simulink model "Lidar_System_July03"  (Simulink 7.3)
settings: Solver=FixedStepDiscrete  StartTime=0.0  StopTime=inf  FixedStep=0.1  MaxStep=0.2  RelTol=1e-3
undefined symbols (not defined in the file): strel
libraries: dspmtrx3 x88, simulink x65, dspstat3 x37, vipstatistics x15, vipmorphops x15, dspindex x1
(part 2 of 8)

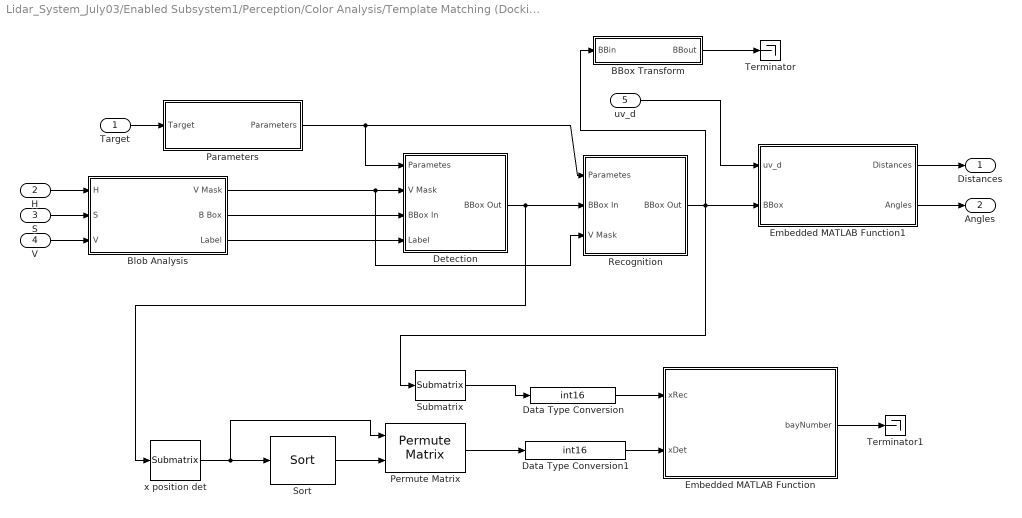
== system Lidar_System_July03/Enabled Subsystem1/Perception/Color Analysis/Template Matching (Docking)/Blue/Circle/Docking1 ==
  Target : Inport
  H : Inport  Port=2
  S : Inport  Port=3
  V : Inport  Port=4
  uv_d : Inport  Port=5
  BBox Transform : Stateflow chart
  Blob Analysis : Subsystem
  Data Type Conversion : DataTypeConversion  OutDataTypeMode=int16  OutDataType=fixdt(1, 16)  OutScaling=2^0  OutDataTypeStr=int16
  Data Type Conversion1 : DataTypeConversion  OutDataTypeMode=int16  OutDataType=fixdt(1, 16)  OutScaling=2^0  OutDataTypeStr=int16
  Detection : Subsystem
  Embedded MATLAB Function : Stateflow chart
  Embedded MATLAB Function1 : Stateflow chart
  Parameters : Subsystem
  Permute Matrix : dspmtrx3/Permute Matrix  mode=Rows  ZeroOneIdxMode=One-based  errmode=Clip index  checkDims=off
  Recognition : Subsystem
  Sort : dspstat3/Sort  DialogController=dspDDGCreate  DialogControllerArgs=DataTag18  otype=Index  dir=Ascending  sortAlg=Quick sort  roundingMode=Floor  overflowMode=off
  Submatrix : dspmtrx3/Submatrix  RowSpan=Range of rows  RowStartMode=First  RowStartIndex=1  RowEndMode=Last  RowEndIndex=1  ColSpan=One column  ColStartMode=First  ColStartIndex=1  ColEndMode=Last  ColEndIndex=1
  Terminator : Terminator
  Terminator1 : Terminator
  x position det : dspmtrx3/Submatrix  RowSpan=Range of rows  RowStartMode=First  RowStartIndex=1  RowEndMode=Last  RowEndIndex=1  ColSpan=One column  ColStartMode=First  ColStartIndex=1  ColEndMode=Last  ColEndIndex=1
  Distances : Outport
  Angles : Outport  Port=2
  wires:
  Embedded MATLAB Function1/2(Angles) -> Angles/1
  BBox Transform/1(BBout) -> Terminator/1
  Target/1 -> Parameters/1(Target)
  V/1 -> Blob Analysis/3(V)
  S/1 -> Blob Analysis/2(S)
  H/1 -> Blob Analysis/1(H)
  Embedded MATLAB Function1/1(Distances) -> Distances/1
  uv_d/1 -> Embedded MATLAB Function1/1(uv_d)
  Embedded MATLAB Function/1(bayNumber) -> Terminator1/1
  Recognition/1(BBox Out) -> BBox Transform/1(BBin), Embedded MATLAB Function1/2(BBox), Submatrix/1
  Data Type Conversion1/1 -> Embedded MATLAB Function/2(xDet)
  Data Type Conversion/1 -> Embedded MATLAB Function/1(xRec)
  Permute Matrix/1 -> Data Type Conversion1/1
  Submatrix/1 -> Data Type Conversion/1
  Sort/1 -> Permute Matrix/2
  x position det/1 -> Permute Matrix/1, Sort/1
  Detection/1(BBox Out) -> x position det/1, Recognition/2(BBox In)
  Blob Analysis/3(Label) -> Detection/4(Label)
  Blob Analysis/2(B Box) -> Detection/3(BBox In)
  Blob Analysis/1(V Mask) -> Recognition/3(V Mask), Detection/2(V Mask)
  Parameters/1(Parameters) -> Recognition/1(Parametes), Detection/1(Parametes)

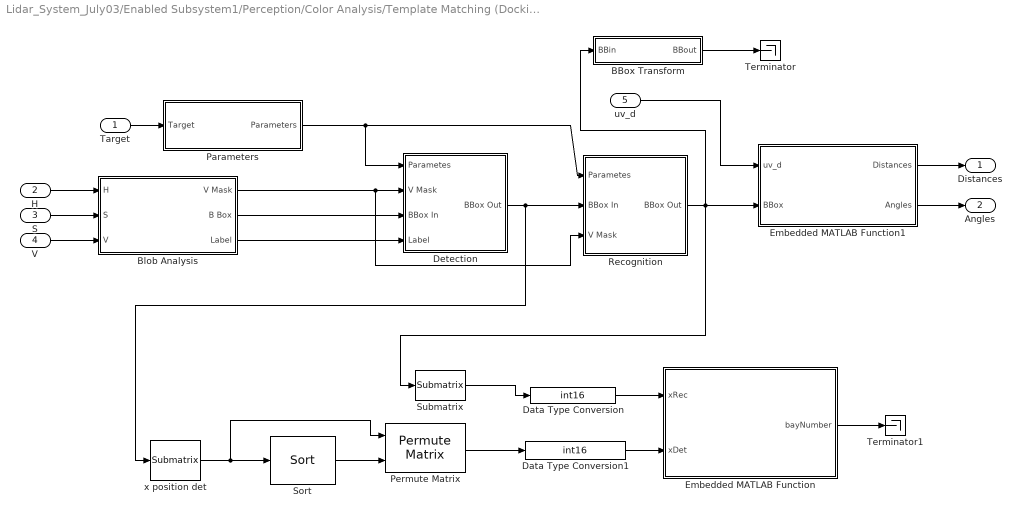
== system Lidar_System_July03/Enabled Subsystem1/Perception/Color Analysis/Template Matching (Docking)/Blue/Cruciform/Docking1 ==
  Target : Inport
  H : Inport  Port=2
  S : Inport  Port=3
  V : Inport  Port=4
  uv_d : Inport  Port=5
  BBox Transform : Stateflow chart
  Blob Analysis : Subsystem
  Data Type Conversion : DataTypeConversion  OutDataTypeMode=int16  OutDataType=fixdt(1, 16)  OutScaling=2^0  OutDataTypeStr=int16
  Data Type Conversion1 : DataTypeConversion  OutDataTypeMode=int16  OutDataType=fixdt(1, 16)  OutScaling=2^0  OutDataTypeStr=int16
  Detection : Subsystem
  Embedded MATLAB Function : Stateflow chart
  Embedded MATLAB Function1 : Stateflow chart
  Parameters : Subsystem
  Permute Matrix : dspmtrx3/Permute Matrix  mode=Rows  ZeroOneIdxMode=One-based  errmode=Clip index  checkDims=off
  Recognition : Subsystem
  Sort : dspstat3/Sort  DialogController=dspDDGCreate  DialogControllerArgs=DataTag22  otype=Index  dir=Ascending  sortAlg=Quick sort  roundingMode=Floor  overflowMode=off
  Submatrix : dspmtrx3/Submatrix  RowSpan=Range of rows  RowStartMode=First  RowStartIndex=1  RowEndMode=Last  RowEndIndex=1  ColSpan=One column  ColStartMode=First  ColStartIndex=1  ColEndMode=Last  ColEndIndex=1
  Terminator : Terminator
  Terminator1 : Terminator
  x position det : dspmtrx3/Submatrix  RowSpan=Range of rows  RowStartMode=First  RowStartIndex=1  RowEndMode=Last  RowEndIndex=1  ColSpan=One column  ColStartMode=First  ColStartIndex=1  ColEndMode=Last  ColEndIndex=1
  Distances : Outport
  Angles : Outport  Port=2
  wires:
  Embedded MATLAB Function1/2(Angles) -> Angles/1
  BBox Transform/1(BBout) -> Terminator/1
  Target/1 -> Parameters/1(Target)
  V/1 -> Blob Analysis/3(V)
  S/1 -> Blob Analysis/2(S)
  H/1 -> Blob Analysis/1(H)
  Embedded MATLAB Function1/1(Distances) -> Distances/1
  uv_d/1 -> Embedded MATLAB Function1/1(uv_d)
  Embedded MATLAB Function/1(bayNumber) -> Terminator1/1
  Recognition/1(BBox Out) -> BBox Transform/1(BBin), Embedded MATLAB Function1/2(BBox), Submatrix/1
  Data Type Conversion1/1 -> Embedded MATLAB Function/2(xDet)
  Data Type Conversion/1 -> Embedded MATLAB Function/1(xRec)
  Permute Matrix/1 -> Data Type Conversion1/1
  Submatrix/1 -> Data Type Conversion/1
  Sort/1 -> Permute Matrix/2
  x position det/1 -> Permute Matrix/1, Sort/1
  Detection/1(BBox Out) -> x position det/1, Recognition/2(BBox In)
  Blob Analysis/3(Label) -> Detection/4(Label)
  Blob Analysis/2(B Box) -> Detection/3(BBox In)
  Blob Analysis/1(V Mask) -> Recognition/3(V Mask), Detection/2(V Mask)
  Parameters/1(Parameters) -> Recognition/1(Parametes), Detection/1(Parametes)

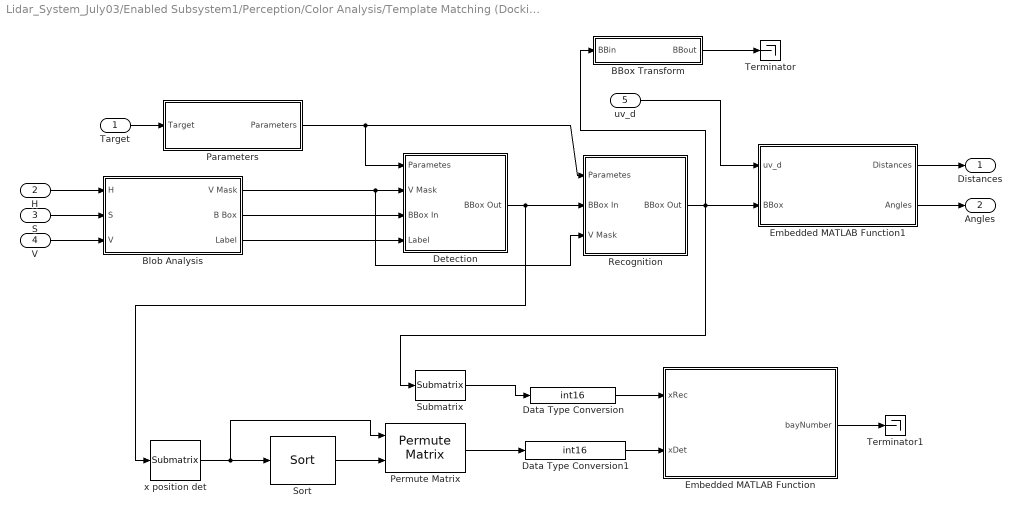
== system Lidar_System_July03/Enabled Subsystem1/Perception/Color Analysis/Template Matching (Docking)/Blue/Triangle/Docking1 ==
  Target : Inport
  H : Inport  Port=2
  S : Inport  Port=3
  V : Inport  Port=4
  uv_d : Inport  Port=5
  BBox Transform : Stateflow chart
  Blob Analysis : Subsystem
  Data Type Conversion : DataTypeConversion  OutDataTypeMode=int16  OutDataType=fixdt(1, 16)  OutScaling=2^0  OutDataTypeStr=int16
  Data Type Conversion1 : DataTypeConversion  OutDataTypeMode=int16  OutDataType=fixdt(1, 16)  OutScaling=2^0  OutDataTypeStr=int16
  Detection : Subsystem
  Embedded MATLAB Function : Stateflow chart
  Embedded MATLAB Function1 : Stateflow chart
  Parameters : Subsystem
  Permute Matrix : dspmtrx3/Permute Matrix  mode=Rows  ZeroOneIdxMode=One-based  errmode=Clip index  checkDims=off
  Recognition : Subsystem
  Sort : dspstat3/Sort  DialogController=dspDDGCreate  DialogControllerArgs=DataTag26  otype=Index  dir=Ascending  sortAlg=Quick sort  roundingMode=Floor  overflowMode=off
  Submatrix : dspmtrx3/Submatrix  RowSpan=Range of rows  RowStartMode=First  RowStartIndex=1  RowEndMode=Last  RowEndIndex=1  ColSpan=One column  ColStartMode=First  ColStartIndex=1  ColEndMode=Last  ColEndIndex=1
  Terminator : Terminator
  Terminator1 : Terminator
  x position det : dspmtrx3/Submatrix  RowSpan=Range of rows  RowStartMode=First  RowStartIndex=1  RowEndMode=Last  RowEndIndex=1  ColSpan=One column  ColStartMode=First  ColStartIndex=1  ColEndMode=Last  ColEndIndex=1
  Distances : Outport
  Angles : Outport  Port=2
  wires:
  Embedded MATLAB Function1/2(Angles) -> Angles/1
  BBox Transform/1(BBout) -> Terminator/1
  Target/1 -> Parameters/1(Target)
  V/1 -> Blob Analysis/3(V)
  S/1 -> Blob Analysis/2(S)
  H/1 -> Blob Analysis/1(H)
  Embedded MATLAB Function1/1(Distances) -> Distances/1
  uv_d/1 -> Embedded MATLAB Function1/1(uv_d)
  Embedded MATLAB Function/1(bayNumber) -> Terminator1/1
  Recognition/1(BBox Out) -> BBox Transform/1(BBin), Embedded MATLAB Function1/2(BBox), Submatrix/1
  Data Type Conversion1/1 -> Embedded MATLAB Function/2(xDet)
  Data Type Conversion/1 -> Embedded MATLAB Function/1(xRec)
  Permute Matrix/1 -> Data Type Conversion1/1
  Submatrix/1 -> Data Type Conversion/1
  Sort/1 -> Permute Matrix/2
  x position det/1 -> Permute Matrix/1, Sort/1
  Detection/1(BBox Out) -> x position det/1, Recognition/2(BBox In)
  Blob Analysis/3(Label) -> Detection/4(Label)
  Blob Analysis/2(B Box) -> Detection/3(BBox In)
  Blob Analysis/1(V Mask) -> Recognition/3(V Mask), Detection/2(V Mask)
  Parameters/1(Parameters) -> Recognition/1(Parametes), Detection/1(Parametes)

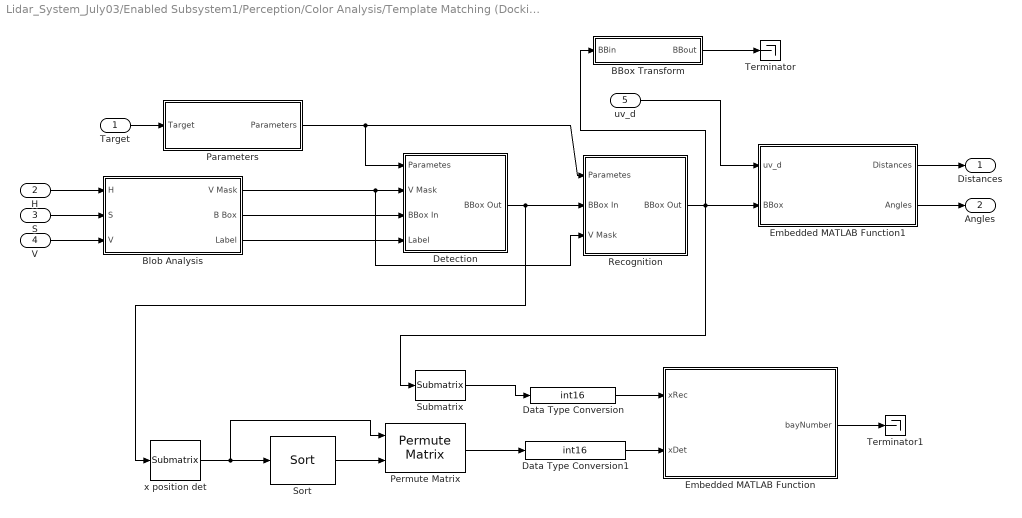
== system Lidar_System_July03/Enabled Subsystem1/Perception/Color Analysis/Template Matching (Docking)/Green/Circle/Docking1 ==
  Target : Inport
  H : Inport  Port=2
  S : Inport  Port=3
  V : Inport  Port=4
  uv_d : Inport  Port=5
  BBox Transform : Stateflow chart
  Blob Analysis : Subsystem
  Data Type Conversion : DataTypeConversion  OutDataTypeMode=int16  OutDataType=fixdt(1, 16)  OutScaling=2^0  OutDataTypeStr=int16
  Data Type Conversion1 : DataTypeConversion  OutDataTypeMode=int16  OutDataType=fixdt(1, 16)  OutScaling=2^0  OutDataTypeStr=int16
  Detection : Subsystem
  Embedded MATLAB Function : Stateflow chart
  Embedded MATLAB Function1 : Stateflow chart
  Parameters : Subsystem
  Permute Matrix : dspmtrx3/Permute Matrix  mode=Rows  ZeroOneIdxMode=One-based  errmode=Clip index  checkDims=off
  Recognition : Subsystem
  Sort : dspstat3/Sort  DialogController=dspDDGCreate  DialogControllerArgs=DataTag30  otype=Index  dir=Ascending  sortAlg=Quick sort  roundingMode=Floor  overflowMode=off
  Submatrix : dspmtrx3/Submatrix  RowSpan=Range of rows  RowStartMode=First  RowStartIndex=1  RowEndMode=Last  RowEndIndex=1  ColSpan=One column  ColStartMode=First  ColStartIndex=1  ColEndMode=Last  ColEndIndex=1
  Terminator : Terminator
  Terminator1 : Terminator
  x position det : dspmtrx3/Submatrix  RowSpan=Range of rows  RowStartMode=First  RowStartIndex=1  RowEndMode=Last  RowEndIndex=1  ColSpan=One column  ColStartMode=First  ColStartIndex=1  ColEndMode=Last  ColEndIndex=1
  Distances : Outport
  Angles : Outport  Port=2
  wires:
  Embedded MATLAB Function1/2(Angles) -> Angles/1
  BBox Transform/1(BBout) -> Terminator/1
  Target/1 -> Parameters/1(Target)
  V/1 -> Blob Analysis/3(V)
  S/1 -> Blob Analysis/2(S)
  H/1 -> Blob Analysis/1(H)
  Embedded MATLAB Function1/1(Distances) -> Distances/1
  uv_d/1 -> Embedded MATLAB Function1/1(uv_d)
  Embedded MATLAB Function/1(bayNumber) -> Terminator1/1
  Recognition/1(BBox Out) -> BBox Transform/1(BBin), Embedded MATLAB Function1/2(BBox), Submatrix/1
  Data Type Conversion1/1 -> Embedded MATLAB Function/2(xDet)
  Data Type Conversion/1 -> Embedded MATLAB Function/1(xRec)
  Permute Matrix/1 -> Data Type Conversion1/1
  Submatrix/1 -> Data Type Conversion/1
  Sort/1 -> Permute Matrix/2
  x position det/1 -> Permute Matrix/1, Sort/1
  Detection/1(BBox Out) -> x position det/1, Recognition/2(BBox In)
  Blob Analysis/3(Label) -> Detection/4(Label)
  Blob Analysis/2(B Box) -> Detection/3(BBox In)
  Blob Analysis/1(V Mask) -> Recognition/3(V Mask), Detection/2(V Mask)
  Parameters/1(Parameters) -> Recognition/1(Parametes), Detection/1(Parametes)

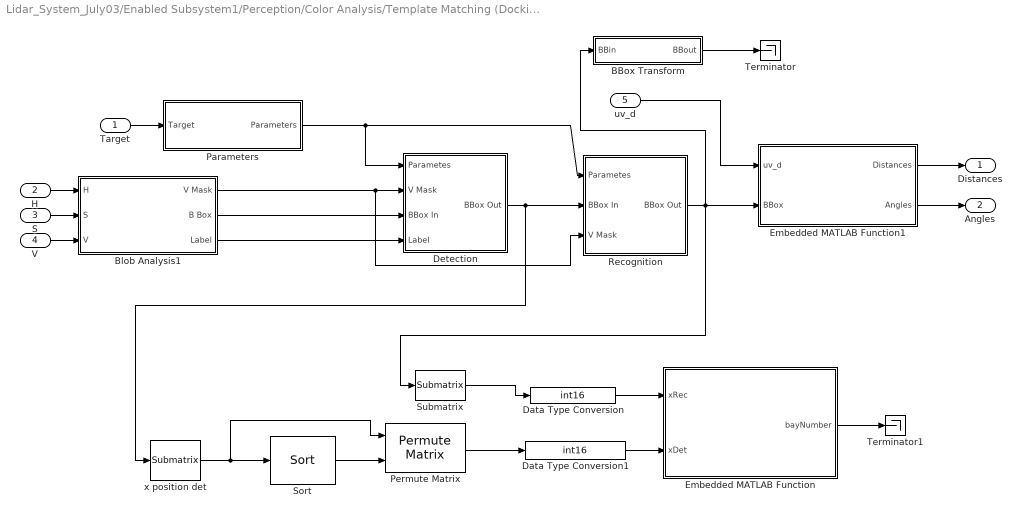
== system Lidar_System_July03/Enabled Subsystem1/Perception/Color Analysis/Template Matching (Docking)/Green/Cruciform/Docking1 ==
  Target : Inport
  H : Inport  Port=2
  S : Inport  Port=3
  V : Inport  Port=4
  uv_d : Inport  Port=5
  BBox Transform : Stateflow chart
  Blob Analysis1 : Subsystem
  Data Type Conversion : DataTypeConversion  OutDataTypeMode=int16  OutDataType=fixdt(1, 16)  OutScaling=2^0  OutDataTypeStr=int16
  Data Type Conversion1 : DataTypeConversion  OutDataTypeMode=int16  OutDataType=fixdt(1, 16)  OutScaling=2^0  OutDataTypeStr=int16
  Detection : Subsystem
  Embedded MATLAB Function : Stateflow chart
  Embedded MATLAB Function1 : Stateflow chart
  Parameters : Subsystem
  Permute Matrix : dspmtrx3/Permute Matrix  mode=Rows  ZeroOneIdxMode=One-based  errmode=Clip index  checkDims=off
  Recognition : Subsystem
  Sort : dspstat3/Sort  DialogController=dspDDGCreate  DialogControllerArgs=DataTag34  otype=Index  dir=Ascending  sortAlg=Quick sort  roundingMode=Floor  overflowMode=off
  Submatrix : dspmtrx3/Submatrix  RowSpan=Range of rows  RowStartMode=First  RowStartIndex=1  RowEndMode=Last  RowEndIndex=1  ColSpan=One column  ColStartMode=First  ColStartIndex=1  ColEndMode=Last  ColEndIndex=1
  Terminator : Terminator
  Terminator1 : Terminator
  x position det : dspmtrx3/Submatrix  RowSpan=Range of rows  RowStartMode=First  RowStartIndex=1  RowEndMode=Last  RowEndIndex=1  ColSpan=One column  ColStartMode=First  ColStartIndex=1  ColEndMode=Last  ColEndIndex=1
  Distances : Outport
  Angles : Outport  Port=2
  wires:
  Embedded MATLAB Function1/2(Angles) -> Angles/1
  BBox Transform/1(BBout) -> Terminator/1
  Target/1 -> Parameters/1(Target)
  V/1 -> Blob Analysis1/3(V)
  S/1 -> Blob Analysis1/2(S)
  H/1 -> Blob Analysis1/1(H)
  Embedded MATLAB Function1/1(Distances) -> Distances/1
  uv_d/1 -> Embedded MATLAB Function1/1(uv_d)
  Embedded MATLAB Function/1(bayNumber) -> Terminator1/1
  Recognition/1(BBox Out) -> BBox Transform/1(BBin), Embedded MATLAB Function1/2(BBox), Submatrix/1
  Data Type Conversion1/1 -> Embedded MATLAB Function/2(xDet)
  Data Type Conversion/1 -> Embedded MATLAB Function/1(xRec)
  Permute Matrix/1 -> Data Type Conversion1/1
  Submatrix/1 -> Data Type Conversion/1
  Sort/1 -> Permute Matrix/2
  x position det/1 -> Permute Matrix/1, Sort/1
  Detection/1(BBox Out) -> x position det/1, Recognition/2(BBox In)
  Blob Analysis1/3(Label) -> Detection/4(Label)
  Blob Analysis1/2(B Box) -> Detection/3(BBox In)
  Blob Analysis1/1(V Mask) -> Recognition/3(V Mask), Detection/2(V Mask)
  Parameters/1(Parameters) -> Recognition/1(Parametes), Detection/1(Parametes)

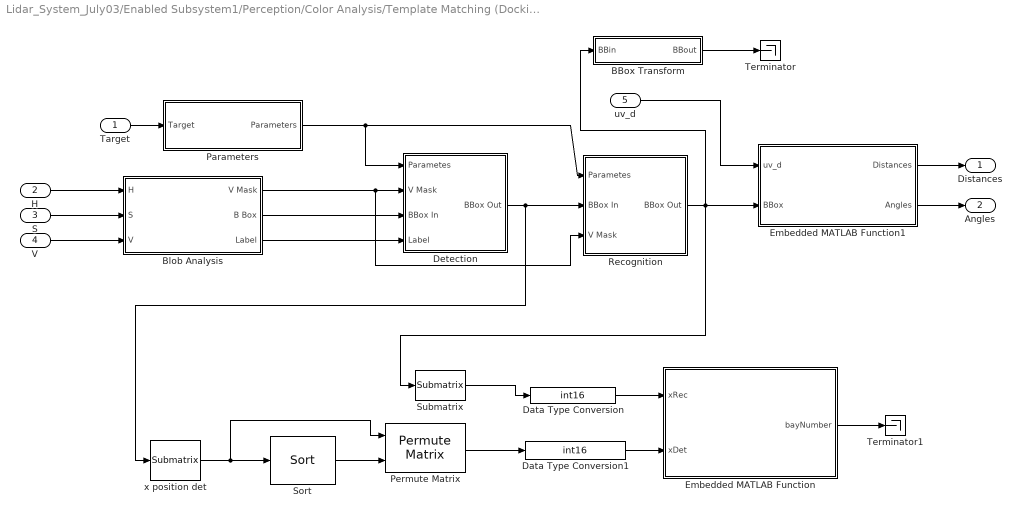
== system Lidar_System_July03/Enabled Subsystem1/Perception/Color Analysis/Template Matching (Docking)/Green/Triangle/Docking1 ==
  Target : Inport
  H : Inport  Port=2
  S : Inport  Port=3
  V : Inport  Port=4
  uv_d : Inport  Port=5
  BBox Transform : Stateflow chart
  Blob Analysis : Subsystem
  Data Type Conversion : DataTypeConversion  OutDataTypeMode=int16  OutDataType=fixdt(1, 16)  OutScaling=2^0  OutDataTypeStr=int16
  Data Type Conversion1 : DataTypeConversion  OutDataTypeMode=int16  OutDataType=fixdt(1, 16)  OutScaling=2^0  OutDataTypeStr=int16
  Detection : Subsystem
  Embedded MATLAB Function : Stateflow chart
  Embedded MATLAB Function1 : Stateflow chart
  Parameters : Subsystem
  Permute Matrix : dspmtrx3/Permute Matrix  mode=Rows  ZeroOneIdxMode=One-based  errmode=Clip index  checkDims=off
  Recognition : Subsystem
  Sort : dspstat3/Sort  DialogController=dspDDGCreate  DialogControllerArgs=DataTag38  otype=Index  dir=Ascending  sortAlg=Quick sort  roundingMode=Floor  overflowMode=off
  Submatrix : dspmtrx3/Submatrix  RowSpan=Range of rows  RowStartMode=First  RowStartIndex=1  RowEndMode=Last  RowEndIndex=1  ColSpan=One column  ColStartMode=First  ColStartIndex=1  ColEndMode=Last  ColEndIndex=1
  Terminator : Terminator
  Terminator1 : Terminator
  x position det : dspmtrx3/Submatrix  RowSpan=Range of rows  RowStartMode=First  RowStartIndex=1  RowEndMode=Last  RowEndIndex=1  ColSpan=One column  ColStartMode=First  ColStartIndex=1  ColEndMode=Last  ColEndIndex=1
  Distances : Outport
  Angles : Outport  Port=2
  wires:
  Embedded MATLAB Function1/2(Angles) -> Angles/1
  BBox Transform/1(BBout) -> Terminator/1
  Target/1 -> Parameters/1(Target)
  V/1 -> Blob Analysis/3(V)
  S/1 -> Blob Analysis/2(S)
  H/1 -> Blob Analysis/1(H)
  Embedded MATLAB Function1/1(Distances) -> Distances/1
  uv_d/1 -> Embedded MATLAB Function1/1(uv_d)
  Embedded MATLAB Function/1(bayNumber) -> Terminator1/1
  Recognition/1(BBox Out) -> BBox Transform/1(BBin), Embedded MATLAB Function1/2(BBox), Submatrix/1
  Data Type Conversion1/1 -> Embedded MATLAB Function/2(xDet)
  Data Type Conversion/1 -> Embedded MATLAB Function/1(xRec)
  Permute Matrix/1 -> Data Type Conversion1/1
  Submatrix/1 -> Data Type Conversion/1
  Sort/1 -> Permute Matrix/2
  x position det/1 -> Permute Matrix/1, Sort/1
  Detection/1(BBox Out) -> x position det/1, Recognition/2(BBox In)
  Blob Analysis/3(Label) -> Detection/4(Label)
  Blob Analysis/2(B Box) -> Detection/3(BBox In)
  Blob Analysis/1(V Mask) -> Recognition/3(V Mask), Detection/2(V Mask)
  Parameters/1(Parameters) -> Recognition/1(Parametes), Detection/1(Parametes)

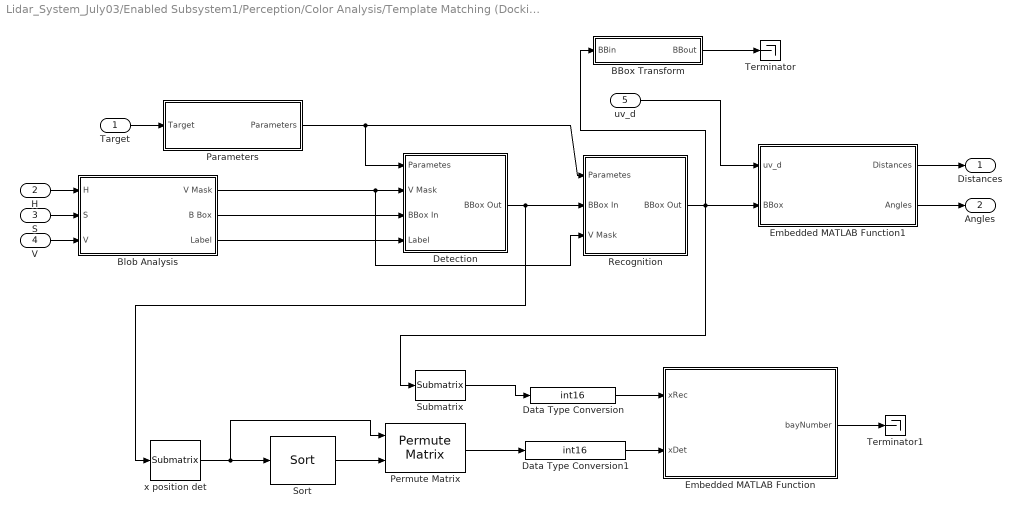
== system Lidar_System_July03/Enabled Subsystem1/Perception/Color Analysis/Template Matching (Docking)/Red/Circle/Docking1 ==
  Target : Inport
  H : Inport  Port=2
  S : Inport  Port=3
  V : Inport  Port=4
  uv_d : Inport  Port=5
  BBox Transform : Stateflow chart
  Blob Analysis : Subsystem
  Data Type Conversion : DataTypeConversion  OutDataTypeMode=int16  OutDataType=fixdt(1, 16)  OutScaling=2^0  OutDataTypeStr=int16
  Data Type Conversion1 : DataTypeConversion  OutDataTypeMode=int16  OutDataType=fixdt(1, 16)  OutScaling=2^0  OutDataTypeStr=int16
  Detection : Subsystem
  Embedded MATLAB Function : Stateflow chart
  Embedded MATLAB Function1 : Stateflow chart
  Parameters : Subsystem
  Permute Matrix : dspmtrx3/Permute Matrix  mode=Rows  ZeroOneIdxMode=One-based  errmode=Clip index  checkDims=off
  Recognition : Subsystem
  Sort : dspstat3/Sort  DialogController=dspDDGCreate  DialogControllerArgs=DataTag42  otype=Index  dir=Ascending  sortAlg=Quick sort  roundingMode=Floor  overflowMode=off
  Submatrix : dspmtrx3/Submatrix  RowSpan=Range of rows  RowStartMode=First  RowStartIndex=1  RowEndMode=Last  RowEndIndex=1  ColSpan=One column  ColStartMode=First  ColStartIndex=1  ColEndMode=Last  ColEndIndex=1
  Terminator : Terminator
  Terminator1 : Terminator
  x position det : dspmtrx3/Submatrix  RowSpan=Range of rows  RowStartMode=First  RowStartIndex=1  RowEndMode=Last  RowEndIndex=1  ColSpan=One column  ColStartMode=First  ColStartIndex=1  ColEndMode=Last  ColEndIndex=1
  Distances : Outport
  Angles : Outport  Port=2
  wires:
  Embedded MATLAB Function1/2(Angles) -> Angles/1
  BBox Transform/1(BBout) -> Terminator/1
  Target/1 -> Parameters/1(Target)
  V/1 -> Blob Analysis/3(V)
  S/1 -> Blob Analysis/2(S)
  H/1 -> Blob Analysis/1(H)
  Embedded MATLAB Function1/1(Distances) -> Distances/1
  uv_d/1 -> Embedded MATLAB Function1/1(uv_d)
  Embedded MATLAB Function/1(bayNumber) -> Terminator1/1
  Recognition/1(BBox Out) -> BBox Transform/1(BBin), Embedded MATLAB Function1/2(BBox), Submatrix/1
  Data Type Conversion1/1 -> Embedded MATLAB Function/2(xDet)
  Data Type Conversion/1 -> Embedded MATLAB Function/1(xRec)
  Permute Matrix/1 -> Data Type Conversion1/1
  Submatrix/1 -> Data Type Conversion/1
  Sort/1 -> Permute Matrix/2
  x position det/1 -> Permute Matrix/1, Sort/1
  Detection/1(BBox Out) -> x position det/1, Recognition/2(BBox In)
  Blob Analysis/3(Label) -> Detection/4(Label)
  Blob Analysis/2(B Box) -> Detection/3(BBox In)
  Blob Analysis/1(V Mask) -> Recognition/3(V Mask), Detection/2(V Mask)
  Parameters/1(Parameters) -> Recognition/1(Parametes), Detection/1(Parametes)

== system Lidar_System_July03/Enabled Subsystem1/Perception/Color Analysis/Template Matching (Docking)/Red/Cruciform/Docking1 ==
  Target : Inport
  H : Inport  Port=2
  S : Inport  Port=3
  V : Inport  Port=4
  uv_d : Inport  Port=5
  BBox Transform : Stateflow chart
  Blob Analysis : Subsystem
  Data Type Conversion : DataTypeConversion  OutDataTypeMode=int16  OutDataType=fixdt(1, 16)  OutScaling=2^0  OutDataTypeStr=int16
  Data Type Conversion1 : DataTypeConversion  OutDataTypeMode=int16  OutDataType=fixdt(1, 16)  OutScaling=2^0  OutDataTypeStr=int16
  Detection : Subsystem
  Embedded MATLAB Function : Stateflow chart
  Embedded MATLAB Function1 : Stateflow chart
  Parameters : Subsystem
  Permute Matrix : dspmtrx3/Permute Matrix  mode=Rows  ZeroOneIdxMode=One-based  errmode=Clip index  checkDims=off
  Recognition : Subsystem
  Sort : dspstat3/Sort  DialogController=dspDDGCreate  DialogControllerArgs=DataTag46  otype=Index  dir=Ascending  sortAlg=Quick sort  roundingMode=Floor  overflowMode=off
  Submatrix : dspmtrx3/Submatrix  RowSpan=Range of rows  RowStartMode=First  RowStartIndex=1  RowEndMode=Last  RowEndIndex=1  ColSpan=One column  ColStartMode=First  ColStartIndex=1  ColEndMode=Last  ColEndIndex=1
  Terminator : Terminator
  Terminator1 : Terminator
  x position det : dspmtrx3/Submatrix  RowSpan=Range of rows  RowStartMode=First  RowStartIndex=1  RowEndMode=Last  RowEndIndex=1  ColSpan=One column  ColStartMode=First  ColStartIndex=1  ColEndMode=Last  ColEndIndex=1
  Distances : Outport
  Angles : Outport  Port=2
  wires:
  Embedded MATLAB Function1/2(Angles) -> Angles/1
  BBox Transform/1(BBout) -> Terminator/1
  Target/1 -> Parameters/1(Target)
  Embedded MATLAB Function1/1(Distances) -> Distances/1
  uv_d/1 -> Embedded MATLAB Function1/1(uv_d)
  Embedded MATLAB Function/1(bayNumber) -> Terminator1/1
  Recognition/1(BBox Out) -> BBox Transform/1(BBin), Embedded MATLAB Function1/2(BBox), Submatrix/1
  Data Type Conversion1/1 -> Embedded MATLAB Function/2(xDet)
  Data Type Conversion/1 -> Embedded MATLAB Function/1(xRec)
  Permute Matrix/1 -> Data Type Conversion1/1
  Submatrix/1 -> Data Type Conversion/1
  Sort/1 -> Permute Matrix/2
  x position det/1 -> Permute Matrix/1, Sort/1
  Detection/1(BBox Out) -> x position det/1, Recognition/2(BBox In)
  Parameters/1(Parameters) -> Recognition/1(Parametes), Detection/1(Parametes)
  V/1 -> Blob Analysis/3(V)
  S/1 -> Blob Analysis/2(S)
  H/1 -> Blob Analysis/1(H)
  Blob Analysis/1(V Mask) -> Detection/2(V Mask), Recognition/3(V Mask)
  Blob Analysis/2(B Box) -> Detection/3(BBox In)
  Blob Analysis/3(Label) -> Detection/4(Label)

== system Lidar_System_July03/Enabled Subsystem1/Perception/Color Analysis/Template Matching (Docking)/Red/Triangle/Docking1 ==
  Target : Inport
  H : Inport  Port=2
  S : Inport  Port=3
  V : Inport  Port=4
  uv_d : Inport  Port=5
  BBox Transform : Stateflow chart
  Blob Analysis : Subsystem
  Data Type Conversion : DataTypeConversion  OutDataTypeMode=int16  OutDataType=fixdt(1, 16)  OutScaling=2^0  OutDataTypeStr=int16
  Data Type Conversion1 : DataTypeConversion  OutDataTypeMode=int16  OutDataType=fixdt(1, 16)  OutScaling=2^0  OutDataTypeStr=int16
  Detection : Subsystem
  Embedded MATLAB Function : Stateflow chart
  Embedded MATLAB Function1 : Stateflow chart
  Parameters : Subsystem
  Permute Matrix : dspmtrx3/Permute Matrix  mode=Rows  ZeroOneIdxMode=One-based  errmode=Clip index  checkDims=off
  Recognition : Subsystem
  Sort : dspstat3/Sort  DialogController=dspDDGCreate  DialogControllerArgs=DataTag50  otype=Index  dir=Ascending  sortAlg=Quick sort  roundingMode=Floor  overflowMode=off
  Submatrix : dspmtrx3/Submatrix  RowSpan=Range of rows  RowStartMode=First  RowStartIndex=1  RowEndMode=Last  RowEndIndex=1  ColSpan=One column  ColStartMode=First  ColStartIndex=1  ColEndMode=Last  ColEndIndex=1
  Terminator : Terminator
  Terminator1 : Terminator
  x position det : dspmtrx3/Submatrix  RowSpan=Range of rows  RowStartMode=First  RowStartIndex=1  RowEndMode=Last  RowEndIndex=1  ColSpan=One column  ColStartMode=First  ColStartIndex=1  ColEndMode=Last  ColEndIndex=1
  Distances : Outport
  Angles : Outport  Port=2
  wires:
  Embedded MATLAB Function1/2(Angles) -> Angles/1
  BBox Transform/1(BBout) -> Terminator/1
  Target/1 -> Parameters/1(Target)
  V/1 -> Blob Analysis/3(V)
  S/1 -> Blob Analysis/2(S)
  H/1 -> Blob Analysis/1(H)
  Embedded MATLAB Function1/1(Distances) -> Distances/1
  uv_d/1 -> Embedded MATLAB Function1/1(uv_d)
  Embedded MATLAB Function/1(bayNumber) -> Terminator1/1
  Recognition/1(BBox Out) -> BBox Transform/1(BBin), Embedded MATLAB Function1/2(BBox), Submatrix/1
  Data Type Conversion1/1 -> Embedded MATLAB Function/2(xDet)
  Data Type Conversion/1 -> Embedded MATLAB Function/1(xRec)
  Permute Matrix/1 -> Data Type Conversion1/1
  Submatrix/1 -> Data Type Conversion/1
  Sort/1 -> Permute Matrix/2
  x position det/1 -> Permute Matrix/1, Sort/1
  Detection/1(BBox Out) -> x position det/1, Recognition/2(BBox In)
  Blob Analysis/3(Label) -> Detection/4(Label)
  Blob Analysis/2(B Box) -> Detection/3(BBox In)
  Blob Analysis/1(V Mask) -> Recognition/3(V Mask), Detection/2(V Mask)
  Parameters/1(Parameters) -> Recognition/1(Parametes), Detection/1(Parametes)

== system Lidar_System_July03/Enabled Subsystem1/Perception/Color Analysis/Template Matching (Docking)/Black/Circle/Docking1/Blob Analysis ==
  H : Inport  OutDataType=fixdt(1, 16)  OutScaling=2^0
  S : Inport  Port=2  OutDataType=fixdt(1, 16)  OutScaling=2^0
  V : Inport  Port=3  OutDataType=fixdt(1, 16)  OutScaling=2^0
  BBox Transform : Stateflow chart  TreatAsAtomicUnit=on
  Blob Analysis : vipstatistics/Blob Analysis  Tag=vipblks_row_conv  DialogController=vipDDGCreate  DialogControllerArgs=DataTag3  area=off  centroid=off  bBox=on  majorAxis=off  minorAxis=off  angle=off  eccentricity=off  equivDiameterSq=off  extent=off  perimeter=off  maxBlobs=10  warnIfNumBlobsExceeded=on  isCount=off  useMinArea=on  minArea=400  useMaxArea=off  maxArea=intmax('uint32')  excludeBorderBlob=on  outDT=double  isOutVarDim=off  isFill=on  fillValues=-1  conn=8  isLabel=on  outputMode=Binary point scaling  outputWordLength=32  outputFracLength=16  firstCoeffMode=Binary point scaling  firstCoeffWordLength=16  firstCoeffFracLength=14  secondCoeffMode=Binary point scaling  secondCoeffWordLength=32  secondCoeffFracLength=16  accumMode=Binary point scaling  accumWordLength=32  accumFracLength=0  prodOutputMode=Binary point scaling  prodOutputWordLength=32  prodOutputFracLength=16  roundingMode=Floor  overflowMode=off
  Closing : vipmorphops/Closing  nhoodsrc=Specify via dialog  strel=strel('disk',1,8)
  Compare To Constant : simulink/Logic and Bit Operations/Compare To Constant  SystemSampleTime=-1  relop=<=  const=70  LogicOutDataTypeMode=boolean  ZeroCross=off
  Terminator : Terminator
  Terminator1 : Terminator
  V Mask : Outport  OutDataType=fixdt(1, 16)  OutScaling=2^0
  B Box : Outport  Port=2  OutDataType=fixdt(1, 16)  OutScaling=2^0
  Label : Outport  Port=3  OutDataType=fixdt(1, 16)  OutScaling=2^0
  wires:
  Compare To Constant/1 -> Closing/1
  H/1 -> Terminator/1
  S/1 -> Terminator1/1
  V/1 -> Compare To Constant/1
  BBox Transform/1(BBout) -> B Box/1
  Closing/1 -> V Mask/1, Blob Analysis/1
  Blob Analysis/1 -> BBox Transform/1(BBin)
  Blob Analysis/2 -> Label/1

== system Lidar_System_July03/Enabled Subsystem1/Perception/Color Analysis/Template Matching (Docking)/Black/Circle/Docking1/Detection ==
  Parametes : Inport  OutDataType=fixdt(1, 16)  OutScaling=2^0
  V Mask : Inport  Port=2  OutDataType=fixdt(1, 16)  OutScaling=2^0
  BBox In : Inport  Port=3  OutDataType=fixdt(1, 16)  OutScaling=2^0
  Label : Inport  Port=4  OutDataType=fixdt(1, 16)  OutScaling=2^0
  Bus Selector : BusSelector  OutputSignals=Templates.Cruciform,Templates.Circle,Templates.Triangle,White Pix Count,Threshold
  Detection : Stateflow chart
  Subsystem : Subsystem
  BBox Out : Outport  OutDataType=fixdt(1, 16)  OutScaling=2^0
  wires:
  Subsystem/1(BBox out) -> BBox Out/1
  Detection/1(bbox_out) -> Subsystem/1(BBox in)
  Detection/2(rtnRatioDiff) -> Subsystem/2(Idx)
  Label/1 -> Detection/8(label)
  BBox In/1 -> Detection/7(bbox_in)
  V Mask/1 -> Detection/6(V_mask)
  Bus Selector/5 -> Detection/5(threshold)  "<Threshold>"
  Bus Selector/4 -> Detection/4(whitePixCount)  "<White Pix Count>"
  Bus Selector/3 -> Detection/3(triangle)  "<Triangle>"
  Bus Selector/2 -> Detection/2(circle)  "<Circle>"
  Bus Selector/1 -> Detection/1(cruciform)  "<Cruciform>"
  Parametes/1 -> Bus Selector/1

== system Lidar_System_July03/Enabled Subsystem1/Perception/Color Analysis/Template Matching (Docking)/Black/Circle/Docking1/Parameters ==
  Target : Inport
  Bus Creator : BusCreator
  Ratio Difference Threshold : Constant  Value=0.6  OutDataType=fixdt(1, 16)  OutScaling=2^0
  Templates : Subsystem
  White Pixel Count : Constant  Value="[144\t64\t180]"  OutDataType=fixdt(1, 16)  OutScaling=2^0
  Parameters : Outport  OutDataType=fixdt(1, 16)  OutScaling=2^0
  wires:
  Bus Creator/1 -> Parameters/1
  Ratio Difference Threshold/1 -> Bus Creator/4  "Threshold"
  White Pixel Count/1 -> Bus Creator/3  "White Pix Count"
  Templates/1(Templates) -> Bus Creator/2  "Templates"
  Target/1 -> Bus Creator/1  "Target Template"

== system Lidar_System_July03/Enabled Subsystem1/Perception/Color Analysis/Template Matching (Docking)/Black/Circle/Docking1/Recognition ==
  Parametes : Inport  OutDataType=fixdt(1, 16)  OutScaling=2^0
  BBox In : Inport  Port=2  OutDataType=fixdt(1, 16)  OutScaling=2^0
  V Mask : Inport  Port=3  OutDataType=fixdt(1, 16)  OutScaling=2^0
  Bus Selector : BusSelector  OutputSignals=Target Template,Templates.Cruciform,Templates.Circle,Templates.Triangle,White Pix Count,Threshold
  Embedded MATLAB Function : Stateflow chart
  Subsystem : Subsystem
  BBox Out : Outport  OutDataType=fixdt(1, 16)  OutScaling=2^0
  wires:
  Embedded MATLAB Function/2(returnRatioDiff) -> Subsystem/2(Idx)
  Embedded MATLAB Function/1(bbox_out) -> Subsystem/1(BBox in)
  BBox In/1 -> Embedded MATLAB Function/8(bbox_in)
  V Mask/1 -> Embedded MATLAB Function/7(V_mask)
  Bus Selector/6 -> Embedded MATLAB Function/6(threshold)  "<Threshold>"
  Bus Selector/5 -> Embedded MATLAB Function/5(whitePixCount)  "<White Pix Count>"
  Bus Selector/4 -> Embedded MATLAB Function/4(triangle)  "<Triangle>"
  Bus Selector/3 -> Embedded MATLAB Function/3(circle)  "<Circle>"
  Bus Selector/2 -> Embedded MATLAB Function/2(cruciform)  "<Cruciform>"
  Bus Selector/1 -> Embedded MATLAB Function/1(targetTemp)  "<Target Template>"
  Parametes/1 -> Bus Selector/1
  Subsystem/1(BBox out) -> BBox Out/1

== system Lidar_System_July03/Enabled Subsystem1/Perception/Color Analysis/Template Matching (Docking)/Black/Cruciform/Docking1/Blob Analysis ==
  H : Inport  OutDataType=fixdt(1, 16)  OutScaling=2^0
  S : Inport  Port=2  OutDataType=fixdt(1, 16)  OutScaling=2^0
  V : Inport  Port=3  OutDataType=fixdt(1, 16)  OutScaling=2^0
  BBox Transform : Stateflow chart  TreatAsAtomicUnit=on
  Blob Analysis : vipstatistics/Blob Analysis  Tag=vipblks_row_conv  DialogController=vipDDGCreate  DialogControllerArgs=DataTag7  area=off  centroid=off  bBox=on  majorAxis=off  minorAxis=off  angle=off  eccentricity=off  equivDiameterSq=off  extent=off  perimeter=off  maxBlobs=10  warnIfNumBlobsExceeded=on  isCount=off  useMinArea=on  minArea=400  useMaxArea=off  maxArea=intmax('uint32')  excludeBorderBlob=on  outDT=double  isOutVarDim=off  isFill=on  fillValues=-1  conn=8  isLabel=on  outputMode=Binary point scaling  outputWordLength=32  outputFracLength=16  firstCoeffMode=Binary point scaling  firstCoeffWordLength=16  firstCoeffFracLength=14  secondCoeffMode=Binary point scaling  secondCoeffWordLength=32  secondCoeffFracLength=16  accumMode=Binary point scaling  accumWordLength=32  accumFracLength=0  prodOutputMode=Binary point scaling  prodOutputWordLength=32  prodOutputFracLength=16  roundingMode=Floor  overflowMode=off
  Closing : vipmorphops/Closing  nhoodsrc=Specify via dialog  strel=strel('disk',1,8)
  Compare To Constant : simulink/Logic and Bit Operations/Compare To Constant  SystemSampleTime=-1  relop=<=  const=70  LogicOutDataTypeMode=boolean  ZeroCross=off
  Terminator : Terminator
  Terminator1 : Terminator
  V Mask : Outport  OutDataType=fixdt(1, 16)  OutScaling=2^0
  B Box : Outport  Port=2  OutDataType=fixdt(1, 16)  OutScaling=2^0
  Label : Outport  Port=3  OutDataType=fixdt(1, 16)  OutScaling=2^0
  wires:
  Compare To Constant/1 -> Closing/1
  H/1 -> Terminator/1
  S/1 -> Terminator1/1
  V/1 -> Compare To Constant/1
  BBox Transform/1(BBout) -> B Box/1
  Closing/1 -> V Mask/1, Blob Analysis/1
  Blob Analysis/1 -> BBox Transform/1(BBin)
  Blob Analysis/2 -> Label/1

== system Lidar_System_July03/Enabled Subsystem1/Perception/Color Analysis/Template Matching (Docking)/Black/Cruciform/Docking1/Detection ==
  Parametes : Inport  OutDataType=fixdt(1, 16)  OutScaling=2^0
  V Mask : Inport  Port=2  OutDataType=fixdt(1, 16)  OutScaling=2^0
  BBox In : Inport  Port=3  OutDataType=fixdt(1, 16)  OutScaling=2^0
  Label : Inport  Port=4  OutDataType=fixdt(1, 16)  OutScaling=2^0
  Bus Selector : BusSelector  OutputSignals=Templates.Cruciform,Templates.Circle,Templates.Triangle,White Pix Count,Threshold
  Detection : Stateflow chart
  Subsystem : Subsystem
  BBox Out : Outport  OutDataType=fixdt(1, 16)  OutScaling=2^0
  wires:
  Subsystem/1(BBox out) -> BBox Out/1
  Detection/1(bbox_out) -> Subsystem/1(BBox in)
  Detection/2(rtnRatioDiff) -> Subsystem/2(Idx)
  Label/1 -> Detection/8(label)
  BBox In/1 -> Detection/7(bbox_in)
  V Mask/1 -> Detection/6(V_mask)
  Bus Selector/5 -> Detection/5(threshold)  "<Threshold>"
  Bus Selector/4 -> Detection/4(whitePixCount)  "<White Pix Count>"
  Bus Selector/3 -> Detection/3(triangle)  "<Triangle>"
  Bus Selector/2 -> Detection/2(circle)  "<Circle>"
  Bus Selector/1 -> Detection/1(cruciform)  "<Cruciform>"
  Parametes/1 -> Bus Selector/1

== system Lidar_System_July03/Enabled Subsystem1/Perception/Color Analysis/Template Matching (Docking)/Black/Cruciform/Docking1/Parameters ==
  Target : Inport
  Bus Creator : BusCreator
  Ratio Difference Threshold : Constant  Value=0.6  OutDataType=fixdt(1, 16)  OutScaling=2^0
  Templates : Subsystem
  White Pixel Count : Constant  Value="[144\t64\t180]"  OutDataType=fixdt(1, 16)  OutScaling=2^0
  Parameters : Outport  OutDataType=fixdt(1, 16)  OutScaling=2^0
  wires:
  Bus Creator/1 -> Parameters/1
  Ratio Difference Threshold/1 -> Bus Creator/4  "Threshold"
  White Pixel Count/1 -> Bus Creator/3  "White Pix Count"
  Templates/1(Templates) -> Bus Creator/2  "Templates"
  Target/1 -> Bus Creator/1  "Target Template"

== system Lidar_System_July03/Enabled Subsystem1/Perception/Color Analysis/Template Matching (Docking)/Black/Cruciform/Docking1/Recognition ==
  Parametes : Inport  OutDataType=fixdt(1, 16)  OutScaling=2^0
  BBox In : Inport  Port=2  OutDataType=fixdt(1, 16)  OutScaling=2^0
  V Mask : Inport  Port=3  OutDataType=fixdt(1, 16)  OutScaling=2^0
  Bus Selector : BusSelector  OutputSignals=Target Template,Templates.Cruciform,Templates.Circle,Templates.Triangle,White Pix Count,Threshold
  Embedded MATLAB Function : Stateflow chart
  Subsystem : Subsystem
  BBox Out : Outport  OutDataType=fixdt(1, 16)  OutScaling=2^0
  wires:
  Embedded MATLAB Function/2(returnRatioDiff) -> Subsystem/2(Idx)
  Embedded MATLAB Function/1(bbox_out) -> Subsystem/1(BBox in)
  BBox In/1 -> Embedded MATLAB Function/8(bbox_in)
  V Mask/1 -> Embedded MATLAB Function/7(V_mask)
  Bus Selector/6 -> Embedded MATLAB Function/6(threshold)  "<Threshold>"
  Bus Selector/5 -> Embedded MATLAB Function/5(whitePixCount)  "<White Pix Count>"
  Bus Selector/4 -> Embedded MATLAB Function/4(triangle)  "<Triangle>"
  Bus Selector/3 -> Embedded MATLAB Function/3(circle)  "<Circle>"
  Bus Selector/2 -> Embedded MATLAB Function/2(cruciform)  "<Cruciform>"
  Bus Selector/1 -> Embedded MATLAB Function/1(targetTemp)  "<Target Template>"
  Parametes/1 -> Bus Selector/1
  Subsystem/1(BBox out) -> BBox Out/1

== system Lidar_System_July03/Enabled Subsystem1/Perception/Color Analysis/Template Matching (Docking)/Black/Triangle/Docking1/Blob Analysis ==
  H : Inport  OutDataType=fixdt(1, 16)  OutScaling=2^0
  S : Inport  Port=2  OutDataType=fixdt(1, 16)  OutScaling=2^0
  V : Inport  Port=3  OutDataType=fixdt(1, 16)  OutScaling=2^0
  BBox Transform : Stateflow chart  TreatAsAtomicUnit=on
  Blob Analysis : vipstatistics/Blob Analysis  Tag=vipblks_row_conv  DialogController=vipDDGCreate  DialogControllerArgs=DataTag11  area=off  centroid=off  bBox=on  majorAxis=off  minorAxis=off  angle=off  eccentricity=off  equivDiameterSq=off  extent=off  perimeter=off  maxBlobs=10  warnIfNumBlobsExceeded=on  isCount=off  useMinArea=on  minArea=400  useMaxArea=off  maxArea=intmax('uint32')  excludeBorderBlob=on  outDT=double  isOutVarDim=off  isFill=on  fillValues=-1  conn=8  isLabel=on  outputMode=Binary point scaling  outputWordLength=32  outputFracLength=16  firstCoeffMode=Binary point scaling  firstCoeffWordLength=16  firstCoeffFracLength=14  secondCoeffMode=Binary point scaling  secondCoeffWordLength=32  secondCoeffFracLength=16  accumMode=Binary point scaling  accumWordLength=32  accumFracLength=0  prodOutputMode=Binary point scaling  prodOutputWordLength=32  prodOutputFracLength=16  roundingMode=Floor  overflowMode=off
  Closing : vipmorphops/Closing  nhoodsrc=Specify via dialog  strel=strel('disk',1,8)
  Compare To Constant : simulink/Logic and Bit Operations/Compare To Constant  SystemSampleTime=-1  relop=<=  const=70  LogicOutDataTypeMode=boolean  ZeroCross=off
  Terminator : Terminator
  Terminator1 : Terminator
  V Mask : Outport  OutDataType=fixdt(1, 16)  OutScaling=2^0
  B Box : Outport  Port=2  OutDataType=fixdt(1, 16)  OutScaling=2^0
  Label : Outport  Port=3  OutDataType=fixdt(1, 16)  OutScaling=2^0
  wires:
  Compare To Constant/1 -> Closing/1
  H/1 -> Terminator/1
  S/1 -> Terminator1/1
  V/1 -> Compare To Constant/1
  BBox Transform/1(BBout) -> B Box/1
  Closing/1 -> V Mask/1, Blob Analysis/1
  Blob Analysis/1 -> BBox Transform/1(BBin)
  Blob Analysis/2 -> Label/1

== system Lidar_System_July03/Enabled Subsystem1/Perception/Color Analysis/Template Matching (Docking)/Black/Triangle/Docking1/Detection ==
  Parametes : Inport  OutDataType=fixdt(1, 16)  OutScaling=2^0
  V Mask : Inport  Port=2  OutDataType=fixdt(1, 16)  OutScaling=2^0
  BBox In : Inport  Port=3  OutDataType=fixdt(1, 16)  OutScaling=2^0
  Label : Inport  Port=4  OutDataType=fixdt(1, 16)  OutScaling=2^0
  Bus Selector : BusSelector  OutputSignals=Templates.Cruciform,Templates.Circle,Templates.Triangle,White Pix Count,Threshold
  Detection : Stateflow chart
  Subsystem : Subsystem
  BBox Out : Outport  OutDataType=fixdt(1, 16)  OutScaling=2^0
  wires:
  Subsystem/1(BBox out) -> BBox Out/1
  Detection/1(bbox_out) -> Subsystem/1(BBox in)
  Detection/2(rtnRatioDiff) -> Subsystem/2(Idx)
  Label/1 -> Detection/8(label)
  BBox In/1 -> Detection/7(bbox_in)
  V Mask/1 -> Detection/6(V_mask)
  Bus Selector/5 -> Detection/5(threshold)  "<Threshold>"
  Bus Selector/4 -> Detection/4(whitePixCount)  "<White Pix Count>"
  Bus Selector/3 -> Detection/3(triangle)  "<Triangle>"
  Bus Selector/2 -> Detection/2(circle)  "<Circle>"
  Bus Selector/1 -> Detection/1(cruciform)  "<Cruciform>"
  Parametes/1 -> Bus Selector/1

== system Lidar_System_July03/Enabled Subsystem1/Perception/Color Analysis/Template Matching (Docking)/Black/Triangle/Docking1/Parameters ==
  Target : Inport
  Bus Creator : BusCreator
  Ratio Difference Threshold : Constant  Value=0.6  OutDataType=fixdt(1, 16)  OutScaling=2^0
  Templates : Subsystem
  White Pixel Count : Constant  Value="[144\t64\t180]"  OutDataType=fixdt(1, 16)  OutScaling=2^0
  Parameters : Outport  OutDataType=fixdt(1, 16)  OutScaling=2^0
  wires:
  Bus Creator/1 -> Parameters/1
  Ratio Difference Threshold/1 -> Bus Creator/4  "Threshold"
  White Pixel Count/1 -> Bus Creator/3  "White Pix Count"
  Templates/1(Templates) -> Bus Creator/2  "Templates"
  Target/1 -> Bus Creator/1  "Target Template"

== system Lidar_System_July03/Enabled Subsystem1/Perception/Color Analysis/Template Matching (Docking)/Black/Triangle/Docking1/Recognition ==
  Parametes : Inport  OutDataType=fixdt(1, 16)  OutScaling=2^0
  BBox In : Inport  Port=2  OutDataType=fixdt(1, 16)  OutScaling=2^0
  V Mask : Inport  Port=3  OutDataType=fixdt(1, 16)  OutScaling=2^0
  Bus Selector : BusSelector  OutputSignals=Target Template,Templates.Cruciform,Templates.Circle,Templates.Triangle,White Pix Count,Threshold
  Embedded MATLAB Function : Stateflow chart
  Subsystem : Subsystem
  BBox Out : Outport  OutDataType=fixdt(1, 16)  OutScaling=2^0
  wires:
  Embedded MATLAB Function/2(returnRatioDiff) -> Subsystem/2(Idx)
  Embedded MATLAB Function/1(bbox_out) -> Subsystem/1(BBox in)
  BBox In/1 -> Embedded MATLAB Function/8(bbox_in)
  V Mask/1 -> Embedded MATLAB Function/7(V_mask)
  Bus Selector/6 -> Embedded MATLAB Function/6(threshold)  "<Threshold>"
  Bus Selector/5 -> Embedded MATLAB Function/5(whitePixCount)  "<White Pix Count>"
  Bus Selector/4 -> Embedded MATLAB Function/4(triangle)  "<Triangle>"
  Bus Selector/3 -> Embedded MATLAB Function/3(circle)  "<Circle>"
  Bus Selector/2 -> Embedded MATLAB Function/2(cruciform)  "<Cruciform>"
  Bus Selector/1 -> Embedded MATLAB Function/1(targetTemp)  "<Target Template>"
  Parametes/1 -> Bus Selector/1
  Subsystem/1(BBox out) -> BBox Out/1

== system Lidar_System_July03/Enabled Subsystem1/Perception/Color Analysis/Template Matching (Docking)/Blue/Circle/Docking1/Blob Analysis ==
  H : Inport  OutDataType=fixdt(1, 16)  OutScaling=2^0
  S : Inport  Port=2  OutDataType=fixdt(1, 16)  OutScaling=2^0
  V : Inport  Port=3  OutDataType=fixdt(1, 16)  OutScaling=2^0
  BBox Transform : Stateflow chart
  Blob Analysis : vipstatistics/Blob Analysis  DialogController=vipDDGCreate  DialogControllerArgs=DataTag15  area=off  centroid=off  bBox=on  majorAxis=off  minorAxis=off  angle=off  eccentricity=off  equivDiameterSq=off  extent=off  perimeter=off  maxBlobs=10  warnIfNumBlobsExceeded=on  isCount=off  useMinArea=on  minArea=400  useMaxArea=off  maxArea=intmax('uint32')  excludeBorderBlob=on  outDT=double  isOutVarDim=off  isFill=on  fillValues=-1  conn=8  isLabel=on  outputMode=Binary point scaling  outputWordLength=32  outputFracLength=16  firstCoeffMode=Binary point scaling  firstCoeffWordLength=16  firstCoeffFracLength=14  secondCoeffMode=Binary point scaling  secondCoeffWordLength=32  secondCoeffFracLength=16  accumMode=Binary point scaling  accumWordLength=32  accumFracLength=0  prodOutputMode=Binary point scaling  prodOutputWordLength=32  prodOutputFracLength=16  roundingMode=Floor  overflowMode=off
  Closing : vipmorphops/Closing  nhoodsrc=Specify via dialog  strel=strel('disk',1,8)
  Compare To Constant : simulink/Logic and Bit Operations/Compare To Constant  SystemSampleTime=-1  relop=>=  const=200  LogicOutDataTypeMode=boolean  ZeroCross=off
  Compare To Constant1 : simulink/Logic and Bit Operations/Compare To Constant  SystemSampleTime=-1  relop=<=  const=185  LogicOutDataTypeMode=boolean  ZeroCross=off
  Compare To Constant2 : simulink/Logic and Bit Operations/Compare To Constant  SystemSampleTime=-1  relop=>=  const=110  LogicOutDataTypeMode=boolean  ZeroCross=off
  Compare To Constant3 : simulink/Logic and Bit Operations/Compare To Constant  SystemSampleTime=-1  relop=>=  const=130  LogicOutDataTypeMode=boolean  ZeroCross=off
  Compare To Constant4 : simulink/Logic and Bit Operations/Compare To Constant  SystemSampleTime=-1  relop=<=  const=160  LogicOutDataTypeMode=boolean  ZeroCross=off
  Compare To Constant5 : simulink/Logic and Bit Operations/Compare To Constant  SystemSampleTime=-1  relop=<=  const=255  LogicOutDataTypeMode=boolean  ZeroCross=off
  Logical Operator : Logic  AllPortsSameDT=off  OutDataTypeMode=boolean  LogicDataType=fixdt(0, 8)  OutDataTypeStr=boolean
  Logical Operator1 : Logic  AllPortsSameDT=off  OutDataTypeMode=boolean  LogicDataType=fixdt(0, 8)  OutDataTypeStr=boolean
  Logical Operator2 : Logic  Inputs=3  AllPortsSameDT=off  OutDataTypeMode=boolean  LogicDataType=fixdt(0, 8)  OutDataTypeStr=boolean
  Logical Operator3 : Logic  AllPortsSameDT=off  OutDataTypeMode=boolean  LogicDataType=fixdt(0, 8)  OutDataTypeStr=boolean
  V Mask : Outport  OutDataType=fixdt(1, 16)  OutScaling=2^0
  B Box : Outport  Port=2  OutDataType=fixdt(1, 16)  OutScaling=2^0
  Label : Outport  Port=3  OutDataType=fixdt(1, 16)  OutScaling=2^0
  wires:
  Blob Analysis/2 -> Label/1
  Blob Analysis/1 -> BBox Transform/1(BBin)
  Closing/1 -> Blob Analysis/1, V Mask/1
  BBox Transform/1(BBout) -> B Box/1
  V/1 -> Compare To Constant/1, Compare To Constant5/1
  H/1 -> Compare To Constant2/1, Compare To Constant4/1
  S/1 -> Compare To Constant3/1, Compare To Constant1/1
  Compare To Constant3/1 -> Logical Operator/1
  Compare To Constant1/1 -> Logical Operator/2
  Compare To Constant2/1 -> Logical Operator1/1
  Compare To Constant4/1 -> Logical Operator1/2
  Logical Operator/1 -> Logical Operator2/2
  Logical Operator1/1 -> Logical Operator2/1
  Logical Operator2/1 -> Closing/1
  Compare To Constant5/1 -> Logical Operator3/2
  Compare To Constant/1 -> Logical Operator3/1
  Logical Operator3/1 -> Logical Operator2/3

== system Lidar_System_July03/Enabled Subsystem1/Perception/Color Analysis/Template Matching (Docking)/Blue/Circle/Docking1/Detection ==
  Parametes : Inport  OutDataType=fixdt(1, 16)  OutScaling=2^0
  V Mask : Inport  Port=2  OutDataType=fixdt(1, 16)  OutScaling=2^0
  BBox In : Inport  Port=3  OutDataType=fixdt(1, 16)  OutScaling=2^0
  Label : Inport  Port=4  OutDataType=fixdt(1, 16)  OutScaling=2^0
  Bus Selector : BusSelector  OutputSignals=Templates.Cruciform,Templates.Circle,Templates.Triangle,White Pix Count,Threshold
  Detection : Stateflow chart
  Subsystem : Subsystem
  BBox Out : Outport  OutDataType=fixdt(1, 16)  OutScaling=2^0
  wires:
  Subsystem/1(BBox out) -> BBox Out/1
  Detection/1(bbox_out) -> Subsystem/1(BBox in)
  Detection/2(rtnRatioDiff) -> Subsystem/2(Idx)
  Label/1 -> Detection/8(label)
  BBox In/1 -> Detection/7(bbox_in)
  V Mask/1 -> Detection/6(V_mask)
  Bus Selector/5 -> Detection/5(threshold)  "<Threshold>"
  Bus Selector/4 -> Detection/4(whitePixCount)  "<White Pix Count>"
  Bus Selector/3 -> Detection/3(triangle)  "<Triangle>"
  Bus Selector/2 -> Detection/2(circle)  "<Circle>"
  Bus Selector/1 -> Detection/1(cruciform)  "<Cruciform>"
  Parametes/1 -> Bus Selector/1

== system Lidar_System_July03/Enabled Subsystem1/Perception/Color Analysis/Template Matching (Docking)/Blue/Circle/Docking1/Parameters ==
  Target : Inport
  Bus Creator : BusCreator
  Ratio Difference Threshold : Constant  Value=0.6  OutDataType=fixdt(1, 16)  OutScaling=2^0
  Templates : Subsystem
  White Pixel Count : Constant  Value="[144\t64\t180]"  OutDataType=fixdt(1, 16)  OutScaling=2^0
  Parameters : Outport  OutDataType=fixdt(1, 16)  OutScaling=2^0
  wires:
  Bus Creator/1 -> Parameters/1
  Ratio Difference Threshold/1 -> Bus Creator/4  "Threshold"
  White Pixel Count/1 -> Bus Creator/3  "White Pix Count"
  Templates/1(Templates) -> Bus Creator/2  "Templates"
  Target/1 -> Bus Creator/1  "Target Template"

== system Lidar_System_July03/Enabled Subsystem1/Perception/Color Analysis/Template Matching (Docking)/Blue/Circle/Docking1/Recognition ==
  Parametes : Inport  OutDataType=fixdt(1, 16)  OutScaling=2^0
  BBox In : Inport  Port=2  OutDataType=fixdt(1, 16)  OutScaling=2^0
  V Mask : Inport  Port=3  OutDataType=fixdt(1, 16)  OutScaling=2^0
  Bus Selector : BusSelector  OutputSignals=Target Template,Templates.Cruciform,Templates.Circle,Templates.Triangle,White Pix Count,Threshold
  Embedded MATLAB Function : Stateflow chart
  Subsystem : Subsystem
  BBox Out : Outport  OutDataType=fixdt(1, 16)  OutScaling=2^0
  wires:
  Embedded MATLAB Function/2(returnRatioDiff) -> Subsystem/2(Idx)
  Embedded MATLAB Function/1(bbox_out) -> Subsystem/1(BBox in)
  BBox In/1 -> Embedded MATLAB Function/8(bbox_in)
  V Mask/1 -> Embedded MATLAB Function/7(V_mask)
  Bus Selector/6 -> Embedded MATLAB Function/6(threshold)  "<Threshold>"
  Bus Selector/5 -> Embedded MATLAB Function/5(whitePixCount)  "<White Pix Count>"
  Bus Selector/4 -> Embedded MATLAB Function/4(triangle)  "<Triangle>"
  Bus Selector/3 -> Embedded MATLAB Function/3(circle)  "<Circle>"
  Bus Selector/2 -> Embedded MATLAB Function/2(cruciform)  "<Cruciform>"
  Bus Selector/1 -> Embedded MATLAB Function/1(targetTemp)  "<Target Template>"
  Parametes/1 -> Bus Selector/1
  Subsystem/1(BBox out) -> BBox Out/1
